simulink model "ControlMRAC"  (R2020a)
settings: Solver=FixedStepDiscrete  StartTime=0.0  StopTime=10.0  RelTol=1e-3
model workspace (MAT data in the model file):
  Kd = Simulink.Parameter
  Kd.Value = 0.0008954
  Kd.DataType = 'double'
  Kd.Dimensions = [1 1]
  Ki = Simulink.Parameter
  Ki.Value = 0.39
  Ki.DataType = 'double'
  Ki.Dimensions = [1 1]
  Kp = Simulink.Parameter
  Kp.Value = 0.0121
  Kp.DataType = 'double'
  Kp.Dimensions = [1 1]
  Ts = Simulink.Parameter
  Ts.Value = 0.01
  Ts.DataType = 'double'
  Ts.Dimensions = [1 1]
  a1 = Simulink.Parameter
  a1.Value = -1.805
  a1.DataType = 'auto'
  a1.Dimensions = [1 1]
  a2 = Simulink.Parameter
  a2.Value = 0.8187
  a2.DataType = 'auto'
  a2.Dimensions = [1 1]
  b0 = Simulink.Parameter
  b0.Value = 0.006854
  b0.DataType = 'auto'
  b0.Dimensions = [1 1]
  b1 = Simulink.Parameter
  b1.Value = 0.006412
  b1.DataType = 'auto'
  b1.Dimensions = [1 1]
  gamma = Simulink.Parameter
  gamma.Value = 2.5
  gamma.DataType = 'auto'
  gamma.Dimensions = [1 1]
undefined symbols (not defined in the file): DiscIntNeverNeededParam
libraries: GPIO_Lib x3, TIMERS_Lib x2, USART_Lib x1, simulink x1, STM32_Config_Lib x1
settings Model: OrderedModelArguments=off  Creator=Lenovo  LastModifiedBy=Lenovo
settings OptimizationCC: DefaultParameterBehavior=Inlined  EnhancedBackFolding=on  PassReuseOutputArgsAs=Individual arguments  ZeroExternalMemoryAtStartup=off  ZeroInternalMemoryAtStartup=off  OptimizeBlockOrder=speed  DifferentSizesBufferReuse=on  OptimizationCustomize=off  EfficientTunableParamExpr=on
settings DebuggingCC: MultiTaskDSMMsg=none  ParameterTunabilityLossMsg=error
settings HardwareCC: ProdBitPerPointer=32  ProdBitPerSizeT=32  ProdBitPerPtrDiffT=32  ProdLargestAtomicInteger=Long  ProdWordSize=32  ProdHWDeviceType=STM32CortexM
settings SFSimCC: MATLABDynamicMemAlloc=off
settings RTWCC: Description=stm32 (Embedded Target)  SystemTargetFile=stm32.tlc  TemplateMakefile=stm32.tmf  GenerateReport=on
settings CodeAppCC: ForceParamTrailComments=on  IgnoreCustomStorageClasses=off  MaxIdLength=64  OperatorAnnotations=on  SimulinkDataObjDesc=on  SFDataObjDesc=on  CustomSymbolStrType=$N$R$M  SimulinkBlockComments=off
settings STFCustomTargetCC: TargetLangStandard=C99 (ISO)  CodeReplacementLibrary=ARM CMSIS SIN COS  MultiwordLength=256  ParMdlRefBuildCompliant=on  IncludeMdlTerminateFcn=off  CombineOutputUpdateFcns=on  ERTCustomFileBanners=on  SupportContinuousTime=off  SupportNonInlinedSFcns=off  RemoveResetFunc=on  MATLABClassNameForMDSCustomization=Simulink.SoftwareTarget.ERTCustomization  SystemTargetFile=stm32.tlc
settings ERTTargetCC: TargetLangStandard=C99 (ISO)  CodeReplacementLibrary=ARM CMSIS SIN COS  CompOptLevelCompliant=off  ConcurrentExecutionCompliant=off  IncludeMdlTerminateFcn=off  ModelStepFunctionPrototypeControlCompliant=off  CPPClassGenCompliant=off  UseToolchainInfoCompliant=off  ExtModeStaticAllocSize=256  ExtModeMexFile=ext_serial_win32_comm  ExtModeMexArgs=0,1,115200,10  InlinedParameterPlacement=NonHierarchical  ERTSrcFileBannerTemplate=sourceFileTemplate.cgt  ERTHdrFileBannerTemplate=sourceFileTemplate.cgt  ERTDataSrcFileTemplate=sourceFileTemplate.cgt  ERTDataHdrFileTemplate=sourceFileTemplate.cgt  ERTCustomFileTemplate=customRoutineProcess.tlc

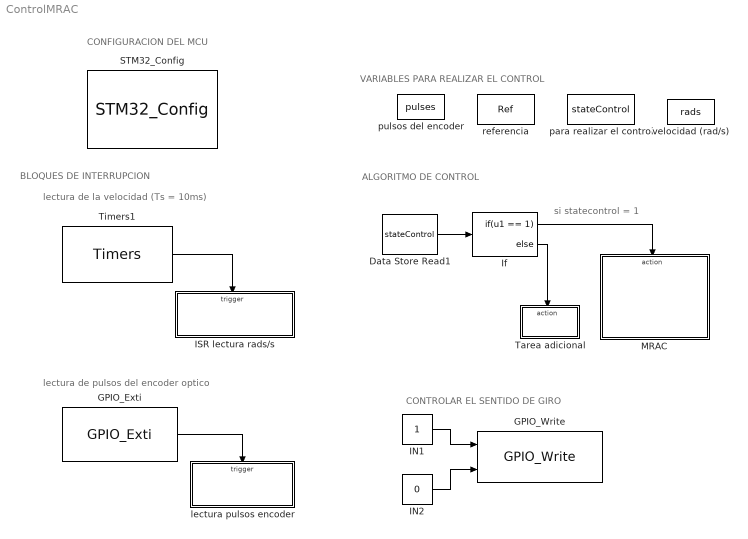
== system ControlMRAC ==
  note: si statecontrol = 1
  note: BLOQUES DE INTERRUPCION
  note: ALGORITMO DE CONTROL
  note: lectura de la velocidad (Ts = 10ms)
  note: lectura de pulsos del encoder optico
  note: CONFIGURACION DEL MCU
  note: CONTROLAR EL SENTIDO DE GIRO
  note: VARIABLES PARA REALIZAR EL CONTROL
  Data Store Read1 : DataStoreRead  DataStoreName=stateControl
  GPIO_Exti : GPIO_Lib/GPIO_Exti  Port_name=GPIOA  Pin_0=on  Pin_1=off  Pin_2=off  Pin_3=off  Pin_4=off  Pin_5=off  Pin_6=off  Pin_7=off  Pin_8=off  Pin_9=off  Pin_10=off  Pin_11=off  Pin_12=off  Pin_13=off  Pin_14=off  Pin_15=off  PinList=GPIOA0
      settings: SourceProductName=Target Support Package - STM32 Adapter
  GPIO_Write : GPIO_Lib/GPIO_Write  Port_name=GPIOB  Pin0=off  Toggle_Pin0=off  Pin1=on  Toggle_Pin1=off  Pin2=off  Toggle_Pin2=off  Pin3=off  Toggle_Pin3=off  Pin4=off  Toggle_Pin4=off  Pin5=off  Toggle_Pin5=off  Pin6=on  Toggle_Pin6=off  Pin7=off  Toggle_Pin7=off  Pin8=off  Toggle_Pin8=off  Pin9=off  Toggle_Pin9=off  Pin10=off  Toggle_Pin10=off  Pin11=off  Toggle_Pin11=off  Pin12=off  Toggle_Pin12=off  Pin13=off  Toggle_Pin13=off  Pin14=off  Toggle_Pin14=off  Pin15=off  Toggle_Pin15=off  PinList="GPIOB1  3  6"
      settings: SourceProductName=Target Support Package - STM32 Adapter
  IN1 : Constant
  IN2 : Constant  Value=0
  ISR lectura rads/s : Subsystem  TreatAsAtomicUnit=on
  If : If  IfExpression=u1 == 1
  MRAC : Subsystem  TreatAsAtomicUnit=on
  STM32_Config : STM32_Config_Lib/STM32_Config  Priority=0  Project_Path=.\  Config_File=ControlMRAC.ioc  MCU_Name=STM32L412KBUx
      settings: SourceProductName=Target Support Package - STM32 Adapter
  Tarea adicional : Subsystem  TreatAsAtomicUnit=on
  Timers1 : TIMERS_Lib/Timers  currentTIM=TIM6  TIM_Name=TIM6  sysUsingTimer=off  TIM_APBClock=80000000  TIM_Set_Clk=off  TIM_Prescaler=79  TIM_Clock=1000000.00  Variable_frequency=off  TIM_Set_OutFreq=off  TIM_ARR=10000  Output_frequency=100.00  Repetition_counter=0  TIM_Mode=Up  TIM_DMA=none  TIM_IRQ=off  TIM_IRQ_ONLY=on  TIM_UP=on  TIM_TRG=off  TIM_COM=off  TIM_BRK=off  NbTIM=2  CH1_enable=off  CH1N_enable=off  CH1_type=Unknown  CH1_DMA=off  CH1_int=off  CH1_edge=Rising  CH1_div=1  CH1_variable_duty=off  CH1_set_pulse=off  CH1_output_duty=0.00  CH1_pulse=0  CH2_enable=off  CH2N_enable=off  CH2_type=Unknown  CH2_DMA=off  CH2_int=off  CH2_edge=Rising  CH2_div=1  CH2_variable_duty=off  CH2_set_pulse=off  CH2_output_duty=0.00  CH2_pulse=0  CH3_enable=off  CH3N_enable=off  CH3_type=Unknown  CH3_DMA=off  CH3_int=off  CH3_edge=Rising  CH3_div=1  CH3_variable_duty=off  CH3_set_pulse=off  CH3_output_duty=0.00  CH3_pulse=0  CH4_enable=off  CH4N_enable=off  CH4_type=Unknown  CH4_DMA=off  CH4_int=off  CH4_edge=Rising  CH4_div=1  CH4_variable_duty=off  CH4_set_pulse=off  CH4_output_duty=0.00  CH4_pulse=0
      settings: SourceProductName=Target Support Package - STM32 Adapter
  "lectura pulsos encoder " : Subsystem  TreatAsAtomicUnit=on
  para realizar el control : DataStoreMemory  DataStoreName=stateControl  ReadBeforeWriteMsg=warning  WriteAfterWriteMsg=warning  WriteAfterReadMsg=warning  ShowAdditionalParam=off
  pulsos del encoder : DataStoreMemory  DataStoreName=pulses  ReadBeforeWriteMsg=warning  WriteAfterWriteMsg=warning  WriteAfterReadMsg=warning  ShowAdditionalParam=off
  referencia : DataStoreMemory  DataStoreName=Ref  ReadBeforeWriteMsg=warning  WriteAfterWriteMsg=warning  WriteAfterReadMsg=warning  ShowAdditionalParam=off
  velocidad (rad/s) : DataStoreMemory  DataStoreName=rads  ReadBeforeWriteMsg=warning  WriteAfterWriteMsg=warning  WriteAfterReadMsg=warning  ShowAdditionalParam=off
  wires:
  Timers1/1 -> ISR lectura rads/s/Trigger
  IN2/1 -> GPIO_Write/2
  IN1/1 -> GPIO_Write/1
  GPIO_Exti/1 -> "lectura pulsos encoder "/Trigger
  Data Store Read1/1 -> If/1
  If/1 -> MRAC/Action
  If/2 -> Tarea adicional/Action

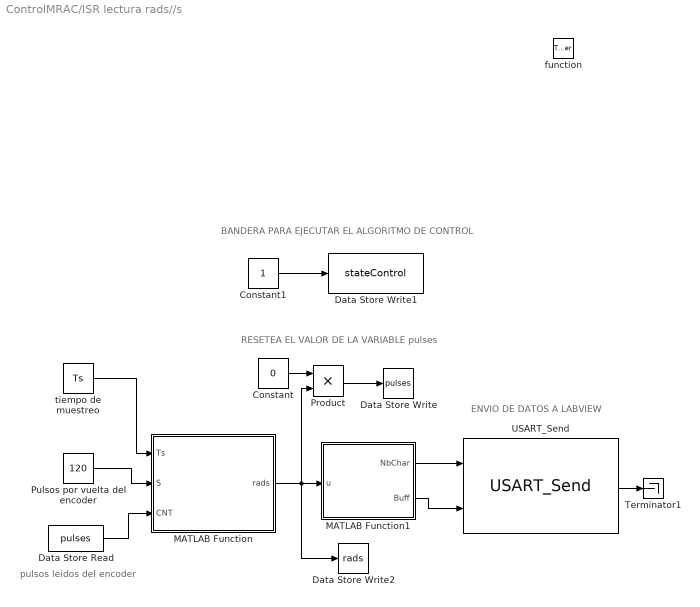
== system ControlMRAC/ISR lectura rads//s ==
  note: pulsos leidos del encoder
  note: BANDERA PARA EJECUTAR EL ALGORITMO DE CONTROL
  note: RESETEA EL VALOR DE LA VARIABLE pulses
  note: ENVIO DE DATOS A LABVIEW
  function : TriggerPort  TriggerType=function-call  VariantControl=Variant
  Constant : Constant  Value=0
  Constant1 : Constant
  Data Store Read : DataStoreRead  DataStoreName=pulses
  Data Store Write : DataStoreWrite  DataStoreName=pulses
  Data Store Write1 : DataStoreWrite  DataStoreName=stateControl
  Data Store Write2 : DataStoreWrite  DataStoreName=rads
  MATLAB Function : MATLAB Function  TreatAsAtomicUnit=on
  MATLAB Function1 : MATLAB Function  TreatAsAtomicUnit=on
  Product : Product
  Pulsos por vuelta del encoder : Constant  Value=120
  Terminator1 : Terminator
  USART_Send : USART_Lib/USART_Send  USART_name=USART2  Buff_size=512  nbUsart=1  usartMode=Asynchronous  usartDma_Rx=off  usartDma_Tx=off  usartIt=on
      settings: SourceProductName=Target Support Package - STM32 Adapter
  tiempo de muestreo : Constant  Value=Ts
  wires:
  Data Store Read/1 -> MATLAB Function/3(CNT)
  Pulsos por vuelta del encoder/1 -> MATLAB Function/2(S)
  tiempo de muestreo/1 -> MATLAB Function/1(Ts)
  MATLAB Function/1(rads) -> Data Store Write2/1, Product/2, MATLAB Function1/1(u)
  MATLAB Function1/2(Buff) -> USART_Send/2
  MATLAB Function1/1(NbChar) -> USART_Send/1
  USART_Send/1 -> Terminator1/1
  Constant/1 -> Product/1
  Product/1 -> Data Store Write/1
  Constant1/1 -> Data Store Write1/1

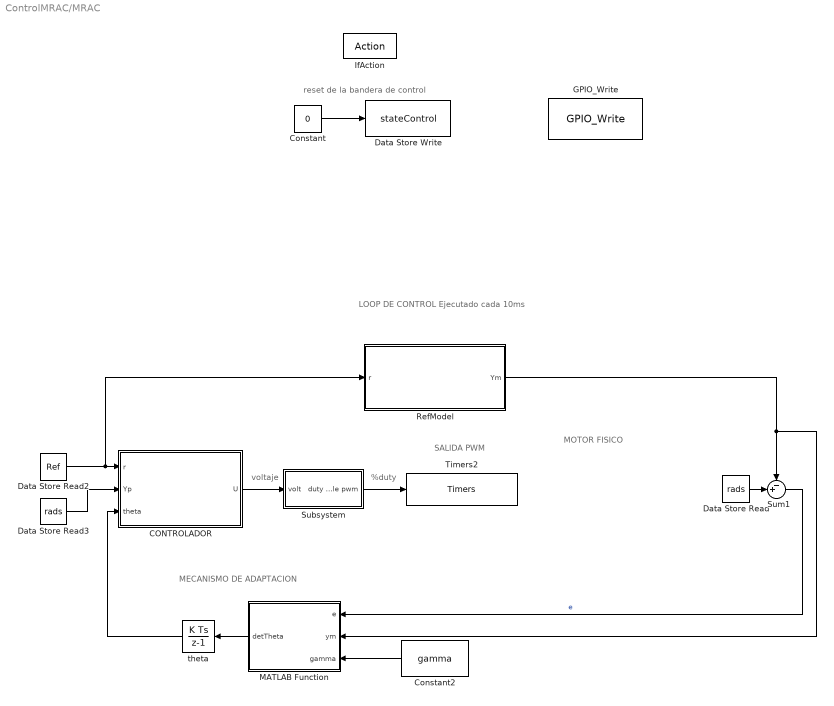
== system ControlMRAC/MRAC ==
  note: MOTOR FISICO
  note: LOOP DE CONTROL
      | Ejecutado cada 10ms
  note: MECANISMO DE ADAPTACION
  note: SALIDA PWM
  note: reset de la bandera de control
  note: %duty
  note: voltaje
  IfAction : ActionPort  ActionPortLabel=if(u1 == 1)
  CONTROLADOR : Subsystem
  Constant : Constant  Value=0
  Constant2 : Constant  Value=gamma
  Data Store Read : DataStoreRead  DataStoreName=rads
  Data Store Read2 : DataStoreRead  DataStoreName=Ref
  Data Store Read3 : DataStoreRead  DataStoreName=rads
  Data Store Write : DataStoreWrite  DataStoreName=stateControl
  GPIO_Write : GPIO_Lib/GPIO_Write  Port_name=GPIOB  Pin0=off  Toggle_Pin0=off  Pin1=off  Toggle_Pin1=off  Pin2=off  Toggle_Pin2=off  Pin3=on  Toggle_Pin3=on  Pin4=off  Toggle_Pin4=off  Pin5=off  Toggle_Pin5=off  Pin6=off  Toggle_Pin6=off  Pin7=off  Toggle_Pin7=off  Pin8=off  Toggle_Pin8=off  Pin9=off  Toggle_Pin9=off  Pin10=off  Toggle_Pin10=off  Pin11=off  Toggle_Pin11=off  Pin12=off  Toggle_Pin12=off  Pin13=off  Toggle_Pin13=off  Pin14=off  Toggle_Pin14=off  Pin15=off  Toggle_Pin15=off  PinList="GPIOB1  3  6"
      settings: SourceProductName=Target Support Package - STM32 Adapter
  MATLAB Function : MATLAB Function  TreatAsAtomicUnit=on
  RefModel : Subsystem
  Subsystem : Subsystem
  Sum1 : Sum  Inputs=-+|
  Timers2 : TIMERS_Lib/Timers  currentTIM=TIM15  TIM_Name=TIM15  sysUsingTimer=off  TIM_APBClock=80000000  TIM_Set_Clk=off  TIM_Prescaler=40-1  TIM_Clock=2000000.00  Variable_frequency=off  TIM_Set_OutFreq=off  TIM_ARR=50  Output_frequency=40000.00  Repetition_counter=0  TIM_Mode=Up  TIM_DMA=none  TIM_IRQ=off  TIM_IRQ_ONLY=on  TIM_UP=off  TIM_TRG=off  TIM_COM=off  TIM_BRK=off  NbTIM=2  CH1_enable=off  CH1N_enable=off  CH1_type=Unknown  CH1_DMA=off  CH1_int=off  CH1_edge=Rising  CH1_div=1  CH1_variable_duty=off  CH1_set_pulse=off  CH1_output_duty=0.00  CH1_pulse=0  CH2_enable=on  CH2N_enable=off  CH2_type=Output_PWM  CH2_DMA=off  CH2_int=off  CH2_edge=Rising  CH2_div=1  CH2_variable_duty=on  CH2_set_pulse=off  CH2_output_duty=0.00  CH2_pulse=0  CH3_enable=off  CH3N_enable=off  CH3_type=Unknown  CH3_DMA=off  CH3_int=off  CH3_edge=Rising  CH3_div=1  CH3_variable_duty=off  CH3_set_pulse=off  CH3_output_duty=0.00  CH3_pulse=0  CH4_enable=off  CH4N_enable=off  CH4_type=Unknown  CH4_DMA=off  CH4_int=off  CH4_edge=Rising  CH4_div=1  CH4_variable_duty=off  CH4_set_pulse=off  CH4_output_duty=0.00  CH4_pulse=0
      settings: SourceProductName=Target Support Package - STM32 Adapter
  theta : DiscreteIntegrator  SampleTime=-1  ICPrevOutput=DiscIntNeverNeededParam  ICPrevScaledInput=DiscIntNeverNeededParam
  wires:
  Constant/1 -> Data Store Write/1
  CONTROLADOR/1(U) -> Subsystem/1(volt)
  Subsystem/1(duty cycle pwm) -> Timers2/1
  Data Store Read2/1 -> RefModel/1(r), CONTROLADOR/1(r)
  Data Store Read3/1 -> CONTROLADOR/2(Yp)
  RefModel/1(Ym) -> MATLAB Function/2(ym), Sum1/1
  Data Store Read/1 -> Sum1/2
  theta/1 -> CONTROLADOR/3(theta)
  MATLAB Function/1(detTheta) -> theta/1
  Sum1/1 -> MATLAB Function/1(e)  "e"
  Constant2/1 -> MATLAB Function/3(gamma)

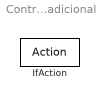
== system ControlMRAC/Tarea adicional ==
  IfAction : ActionPort  ActionPortLabel=else

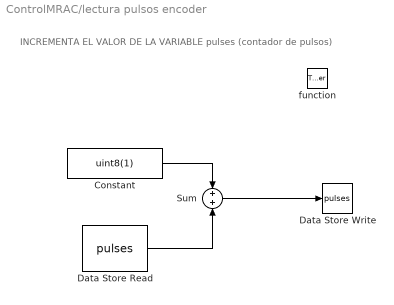
== system ControlMRAC/lectura pulsos encoder  ==
  note: INCREMENTA EL VALOR DE LA VARIABLE pulses (contador de pulsos)
  function : TriggerPort  TriggerType=function-call  VariantControl=Variant
  Constant : Constant  Value=uint8(1)
  Data Store Read : DataStoreRead  DataStoreName=pulses
  Data Store Write : DataStoreWrite  DataStoreName=pulses
  Sum : Sum
  wires:
  Constant/1 -> Sum/1
  Data Store Read/1 -> Sum/2
  Sum/1 -> Data Store Write/1

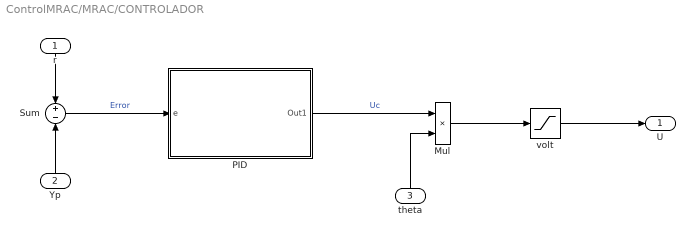
== system ControlMRAC/MRAC/CONTROLADOR ==
  r : Inport
  Yp : Inport  Port=2
  theta : Inport  Port=3
  Mul : Product
  PID : Subsystem
  Sum : Sum  Inputs=+|-
  volt : Saturate  UpperLimit=8.37  LowerLimit=0
  U : Outport  VectorParamsAs1DForOutWhenUnconnected=off
  wires:
  Yp/1 -> Sum/2
  Sum/1 -> PID/1(e)  "Error"
  r/1 -> Sum/1
  PID/1(Out1) -> Mul/1  "Uc"
  theta/1 -> Mul/2
  Mul/1 -> volt/1
  volt/1 -> U/1

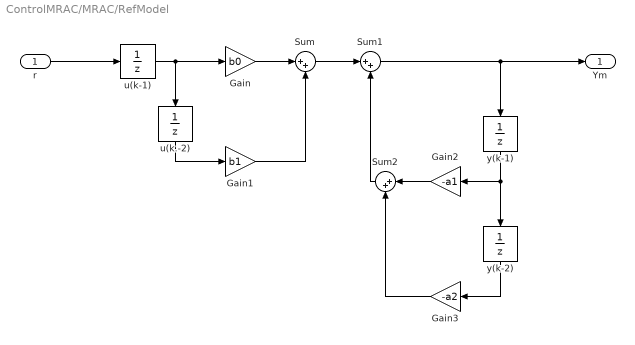
== system ControlMRAC/MRAC/RefModel ==
  r : Inport
  Gain : Gain  Gain=b0
  Gain1 : Gain  Gain=b1
  Gain2 : Gain  Gain=-a1
  Gain3 : Gain  Gain=-a2
  Sum : Sum  Inputs=|++
  Sum1 : Sum  Inputs=|++
  Sum2 : Sum  Inputs=|++
  u(k-1) : UnitDelay  SampleTime=Ts  HasFrameUpgradeWarning=on
  u(k.-2) : UnitDelay  SampleTime=Ts  HasFrameUpgradeWarning=on
  y(k-1) : UnitDelay  SampleTime=Ts  HasFrameUpgradeWarning=on
  y(k-2) : UnitDelay  SampleTime=Ts  HasFrameUpgradeWarning=on
  Ym : Outport
  wires:
  r/1 -> u(k-1)/1
  u(k-1)/1 -> u(k.-2)/1, Gain/1
  Gain/1 -> Sum/1
  u(k.-2)/1 -> Gain1/1
  Gain1/1 -> Sum/2
  Sum/1 -> Sum1/1
  Sum1/1 -> Ym/1, y(k-1)/1
  y(k-1)/1 -> y(k-2)/1, Gain2/1
  y(k-2)/1 -> Gain3/1
  Gain2/1 -> Sum2/1
  Gain3/1 -> Sum2/2
  Sum2/1 -> Sum1/2

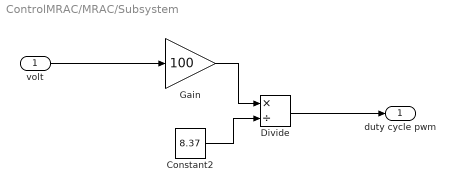
== system ControlMRAC/MRAC/Subsystem ==
  volt : Inport
  Constant2 : Constant  Value=8.37
  Divide : Product  Inputs=*/
  Gain : Gain  Gain=100
  duty cycle pwm : Outport
  wires:
  Constant2/1 -> Divide/2
  Gain/1 -> Divide/1
  volt/1 -> Gain/1
  Divide/1 -> duty cycle pwm/1

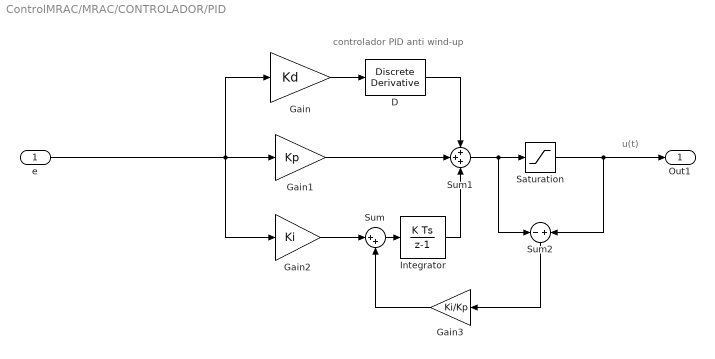
== system ControlMRAC/MRAC/CONTROLADOR/PID ==
  note: controlador PID anti wind-up
  note: u(t)
  e : Inport
  D : simulink/Discrete/Discrete Derivative  gainval=1.0  ICPrevScaledInput=0.0  OutMin=[]  OutMax=[]  OutDataType=fixdt(1, 16)  OutScaling=2^-10  DoSatur=off
  Gain : Gain  Gain=Kd
  Gain1 : Gain  Gain=Kp
  Gain2 : Gain  Gain=Ki
  Gain3 : Gain  Gain=Ki/Kp
  Integrator : DiscreteIntegrator  SampleTime=Ts  ICPrevOutput=DiscIntNeverNeededParam  ICPrevScaledInput=DiscIntNeverNeededParam
  Saturation : Saturate  UpperLimit=8.37  LowerLimit=0
  Sum : Sum  Inputs=|++
  Sum1 : Sum  Inputs=+++
  Sum2 : Sum  Inputs=-+
  Out1 : Outport
  wires:
  Gain1/1 -> Sum1/2
  Sum1/1 -> Sum2/1, Saturation/1
  Gain/1 -> D/1
  Saturation/1 -> Out1/1, Sum2/2
  Sum2/1 -> Gain3/1
  Integrator/1 -> Sum1/3
  Sum/1 -> Integrator/1
  Gain2/1 -> Sum/1
  D/1 -> Sum1/1
  e/1 -> Gain2/1, Gain/1, Gain1/1
  Gain3/1 -> Sum/2

== matlab function ControlMRAC/ISR lectura rads//s/MATLAB Function1 ==
  data: u input; NbChar output; Buff output
function [NbChar, Buff] = convert(u)
if coder.target('Sfun')
    %executing in Matlab, Buff is null
    Buff = uint32(0);
    NbChar = uint16(0);
else
    %executing in the generated code
    buffer = zeros(1,15,'uint8');
%     coder.ceval('sprintf',coder.wref(buffer),['%2.2f',0],u);
%     tmp = uint8(' rad/s');
%     y = [buffer(1:4),tmp,13,10,0];
%     Buff = coder.ceval('getBuffPtr',coder.ref(y));
%     NbChar = uint16(size(y,2));
%     y = [buffer(1:4),13,10,0];
%     Buff = coder.ceval('getBuffPtr',coder.ref(buffer));
%     NbChar = uint16(size(y,2));
    Buff = coder.ceval('getBuffPtr',coder.ref(buffer));
    NbChar = coder.ceval('sprintf',coder.wref(buffer),['%.2f\r\n',0],u);
end

== matlab function ControlMRAC/ISR lectura rads//s/MATLAB Function ==
  data: Ts input; rads output; S input; CNT input
function rads = calc_rads(Ts, S, CNT)
if coder.target('Sfun')
    %executing in Matlab, Buff is null
    rads = double(0);
else
    rpm = CNT * 60.0 / (Ts * S);
    rads = rpm * (2 * pi) / 60;
end

== matlab function ControlMRAC/MRAC/MATLAB Function ==
  data: e input; detTheta output; ym input; gamma input
function detTheta = fcn(e,ym,gamma)
theta0 = 1;
alfa = 35;

detTheta = -gamma *(e*ym/theta0)/(alfa^2 + (ym/theta0)^2)
end
